simulink model "LQR_K_controller"  (R2017b)
settings: Solver=FixedStepAuto  StartTime=0.0  StopTime=inf  RelTol=1e-3
InitFcn:
  | set_kgain_from_physical_model_constraints
undefined symbols (not defined in the file or in its folder): Theta, X, Y
libraries: robotlib x17
settings Model: Creator=apollo  LastModifiedBy=apollo
settings OptimizationCC: PassReuseOutputArgsAs=Individual arguments  MaxStackSize=64
settings DebuggingCC: ParameterTunabilityLossMsg=error
settings HardwareCC: ProdBitPerPointer=32  ProdBitPerSizeT=32  ProdBitPerPtrDiffT=32  ProdLargestAtomicFloat=None  ProdIntDivRoundTo=Undefined  ProdEndianess=Unspecified  ProdWordSize=32  ProdHWDeviceType=Generic->Unspecified (assume 32-bit Generic)  UseEmbeddedCoderFeatures=off
settings SFSimCC: MATLABDynamicMemAlloc=off
settings RTWCC: SystemTargetFile=ert.tlc  HardwareBoard=Robot Operating System (ROS)  GenCodeOnly=on  TemplateMakefile=ert_default_tmf  GenerateReport=on  Toolchain=Catkin  IncludeHyperlinkInReport=on  LaunchReport=on  TargetLang=C++  GenerateTraceInfo=on  GenerateTraceReport=on  GenerateTraceReportSl=on  GenerateTraceReportSf=on  GenerateTraceReportEml=on
settings CodeAppCC: ForceParamTrailComments=on  IgnoreCustomStorageClasses=off  OperatorAnnotations=on  SimulinkDataObjDesc=on  SFDataObjDesc=on  InsertBlockDesc=on
settings ERTTargetCC: SupportNonInlinedSFcns=on

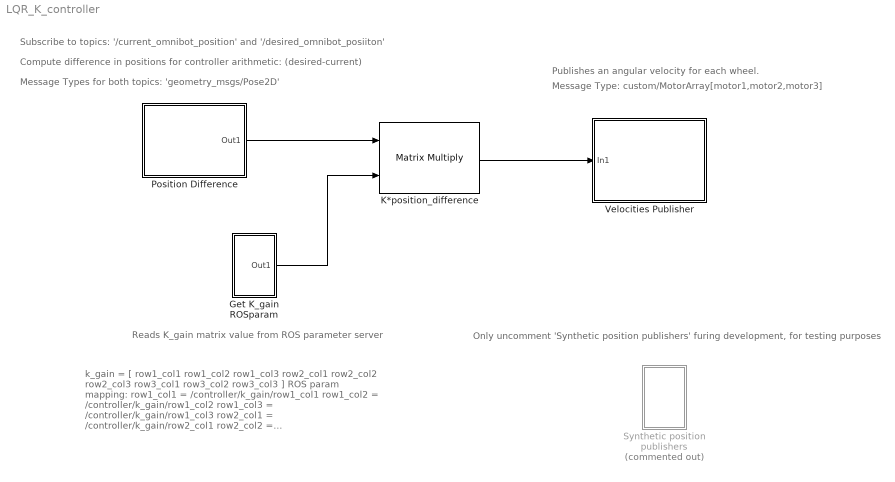
== system LQR_K_controller ==
  note: k_gain = [
      | row1_col1 row1_col2 row1_col3
      | row2_col1 row2_col2 row2_col3
      | row3_col1 row3_col2 row3_col3
      | ]
      |
      | ROS param mapping:
      | row1_col1 = /controller/k_gain/row1_col1
      | row1_col2 = /controller/k_gain/row1_col2
      | row1_col3 = /controller/k_gain/row1_col3
      |
      | row2_col1 = /controller/k_gain/row2_col1
      | row2_col2 = /controller/k_gain/row2_col2
      | row2_col3 = controller/k_gain/row2_col3
      |
      | row3_col1 = /controller/k_gain/row3_col1
      | row3_col2 = /controller/k_gain/row3_col2
      | row3_col3 = /controller/k_gain/row3_col3
  note: Reads K_gain matrix value from ROS parameter server
  note: Publishes an angular velocity for each wheel.
  note: Subscribe to topics: '/current_omnibot_position' and '/desired_omnibot_posiiton'
  note: Only uncomment 'Synthetic position publishers' furing development, for testing purposes
  note: Compute difference in positions for controller arithmetic: (desired-current)
  note: Message Types for both topics: 'geometry_msgs/Pose2D'
  note: Message Type: custom/MotorArray[motor1,motor2,motor3]
  Get K_gain ROSparam : Subsystem
  K*position_difference : Product  Multiplication=Matrix(*)
  Position Difference : Subsystem
  Synthetic position publishers : Subsystem  Commented=on
  Velocities Publisher : Subsystem
  wires:
  K*position_difference/1 -> Velocities Publisher/1(In1)
  Position Difference/1(Out1) -> K*position_difference/1
  Get K_gain ROSparam/1(Out1) -> K*position_difference/2

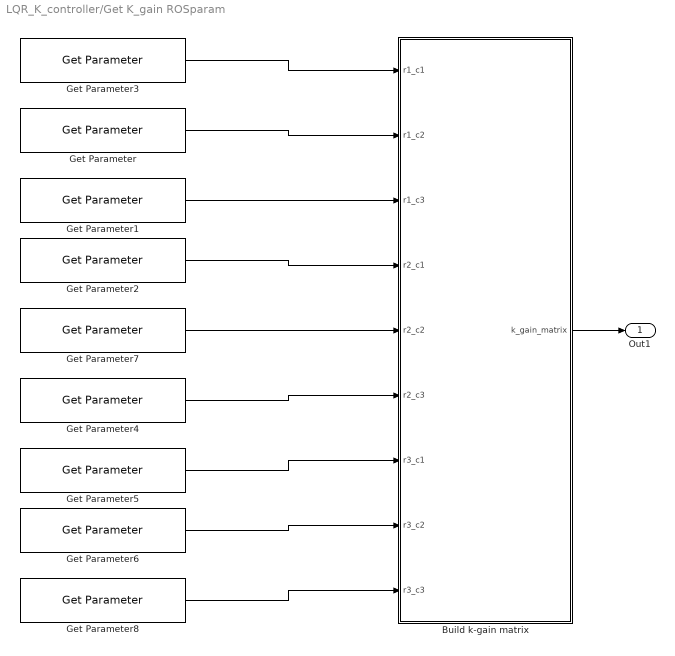
== system LQR_K_controller/Get K_gain ROSparam ==
  Build k-gain matrix : MATLAB Function  TreatAsAtomicUnit=on
  Get Parameter : robotlib/Get Parameter  SourceLibraryInfo=This block requires Robotics System Toolbox  ParameterSource=Specify your own  ParameterName=/controller/k_gain/row1_col2  ParameterType=double  ParameterMaxArrayLength=16  ParameterInitialValue=0.0  SampleTime=-1  ShowErrorCodeOutput=off  ModelName=LQR_K_controller  BlockId=ParamGet_LQR_K_controller_91
      settings: SourceProductName=Robotics System Toolbox  SourceProductBaseCode=RO
  Get Parameter1 : robotlib/Get Parameter  SourceLibraryInfo=This block requires Robotics System Toolbox  ParameterSource=Specify your own  ParameterName=/controller/k_gain/row1_col3  ParameterType=double  ParameterMaxArrayLength=16  ParameterInitialValue=0.0  SampleTime=-1  ShowErrorCodeOutput=off  ModelName=LQR_K_controller  BlockId=ParamGet_LQR_K_controller_92
      settings: SourceProductName=Robotics System Toolbox  SourceProductBaseCode=RO
  Get Parameter2 : robotlib/Get Parameter  SourceLibraryInfo=This block requires Robotics System Toolbox  ParameterSource=Specify your own  ParameterName=/controller/k_gain/row2_col1  ParameterType=double  ParameterMaxArrayLength=16  ParameterInitialValue=0.0  SampleTime=-1  ShowErrorCodeOutput=off  ModelName=LQR_K_controller  BlockId=ParamGet_LQR_K_controller_93
      settings: SourceProductName=Robotics System Toolbox  SourceProductBaseCode=RO
  Get Parameter3 : robotlib/Get Parameter  SourceLibraryInfo=This block requires Robotics System Toolbox  ParameterSource=Specify your own  ParameterName=/controller/k_gain/row1_col1  ParameterType=double  ParameterMaxArrayLength=16  ParameterInitialValue=0.0  SampleTime=-1  ShowErrorCodeOutput=off  ModelName=LQR_K_controller  BlockId=ParamGet_LQR_K_controller_94
      settings: SourceProductName=Robotics System Toolbox  SourceProductBaseCode=RO
  Get Parameter4 : robotlib/Get Parameter  SourceLibraryInfo=This block requires Robotics System Toolbox  ParameterSource=Specify your own  ParameterName=/controller/k_gain/row2_col3  ParameterType=double  ParameterMaxArrayLength=16  ParameterInitialValue=0.0  SampleTime=-1  ShowErrorCodeOutput=off  ModelName=LQR_K_controller  BlockId=ParamGet_LQR_K_controller_95
      settings: SourceProductName=Robotics System Toolbox  SourceProductBaseCode=RO
  Get Parameter5 : robotlib/Get Parameter  SourceLibraryInfo=This block requires Robotics System Toolbox  ParameterSource=Specify your own  ParameterName=/controller/k_gain/row3_col1  ParameterType=double  ParameterMaxArrayLength=16  ParameterInitialValue=0.0  SampleTime=-1  ShowErrorCodeOutput=off  ModelName=LQR_K_controller  BlockId=ParamGet_LQR_K_controller_96
      settings: SourceProductName=Robotics System Toolbox  SourceProductBaseCode=RO
  Get Parameter6 : robotlib/Get Parameter  SourceLibraryInfo=This block requires Robotics System Toolbox  ParameterSource=Specify your own  ParameterName=/controller/k_gain/row3_col2  ParameterType=double  ParameterMaxArrayLength=16  ParameterInitialValue=0.0  SampleTime=-1  ShowErrorCodeOutput=off  ModelName=LQR_K_controller  BlockId=ParamGet_LQR_K_controller_97
      settings: SourceProductName=Robotics System Toolbox  SourceProductBaseCode=RO
  Get Parameter7 : robotlib/Get Parameter  SourceLibraryInfo=This block requires Robotics System Toolbox  ParameterSource=Specify your own  ParameterName=/controller/k_gain/row2_col2  ParameterType=double  ParameterMaxArrayLength=16  ParameterInitialValue=0.0  SampleTime=-1  ShowErrorCodeOutput=off  ModelName=LQR_K_controller  BlockId=ParamGet_LQR_K_controller_98
      settings: SourceProductName=Robotics System Toolbox  SourceProductBaseCode=RO
  Get Parameter8 : robotlib/Get Parameter  SourceLibraryInfo=This block requires Robotics System Toolbox  ParameterSource=Specify your own  ParameterName=/controller/k_gain/row3_col3  ParameterType=double  ParameterMaxArrayLength=16  ParameterInitialValue=0.0  SampleTime=-1  ShowErrorCodeOutput=off  ModelName=LQR_K_controller  BlockId=ParamGet_LQR_K_controller_99
      settings: SourceProductName=Robotics System Toolbox  SourceProductBaseCode=RO
  Out1 : Outport
  wires:
  Get Parameter4/1 -> Build k-gain matrix/6(r2_c3)
  Get Parameter3/1 -> Build k-gain matrix/1(r1_c1)
  Get Parameter/1 -> Build k-gain matrix/2(r1_c2)
  Build k-gain matrix/1(k_gain_matrix) -> Out1/1
  Get Parameter2/1 -> Build k-gain matrix/4(r2_c1)
  Get Parameter7/1 -> Build k-gain matrix/5(r2_c2)
  Get Parameter8/1 -> Build k-gain matrix/9(r3_c3)
  Get Parameter6/1 -> Build k-gain matrix/8(r3_c2)
  Get Parameter5/1 -> Build k-gain matrix/7(r3_c1)
  Get Parameter1/1 -> Build k-gain matrix/3(r1_c3)

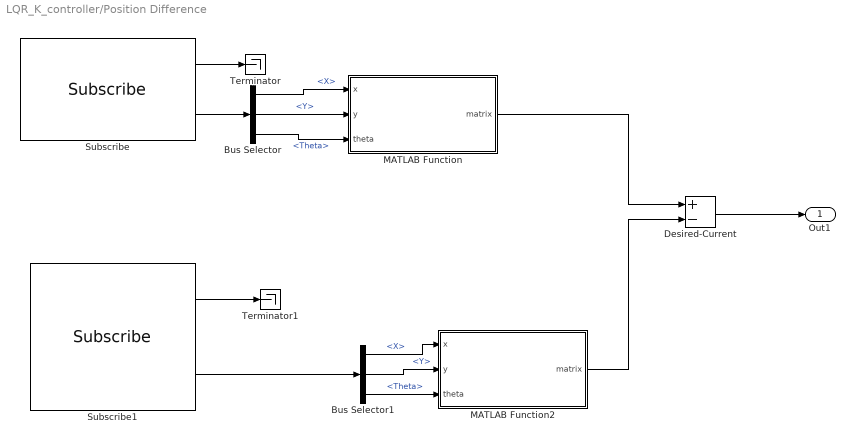
== system LQR_K_controller/Position Difference ==
  Bus Selector : BusSelector  OutputSignals=X,Y,Theta
  Bus Selector1 : BusSelector  OutputSignals=X,Y,Theta
  Desired-Current : Sum  Inputs=+-
  MATLAB Function : MATLAB Function  TreatAsAtomicUnit=on
  MATLAB Function2 : MATLAB Function  TreatAsAtomicUnit=on
  Subscribe : robotlib/Subscribe  SourceLibraryInfo=This block requires Robotics System Toolbox  topicSource=Specify your own  topic=/desired_omnibot_position  messageType=geometry_msgs/Pose2D  sampleTime=-1  messageQueueLength=1
      settings: SourceProductBaseCode=RO
  Subscribe1 : robotlib/Subscribe  SourceLibraryInfo=This block requires Robotics System Toolbox  topicSource=Specify your own  topic=/current_omnibot_position  messageType=geometry_msgs/Pose2D  sampleTime=-1  messageQueueLength=1
      settings: SourceProductBaseCode=RO
  Terminator : Terminator
  Terminator1 : Terminator
  Out1 : Outport
  wires:
  Subscribe/1 -> Terminator/1
  Subscribe1/1 -> Terminator1/1
  Subscribe/2 -> Bus Selector/1
  Bus Selector1/3 -> MATLAB Function2/3(theta)  "<Theta>"
  Bus Selector1/1 -> MATLAB Function2/1(x)  "<X>"
  Bus Selector1/2 -> MATLAB Function2/2(y)  "<Y>"
  Subscribe1/2 -> Bus Selector1/1
  MATLAB Function/1(matrix) -> Desired-Current/1
  Bus Selector/2 -> MATLAB Function/2(y)  "<Y>"
  Bus Selector/1 -> MATLAB Function/1(x)  "<X>"
  Bus Selector/3 -> MATLAB Function/3(theta)  "<Theta>"
  MATLAB Function2/1(matrix) -> Desired-Current/2
  Desired-Current/1 -> Out1/1

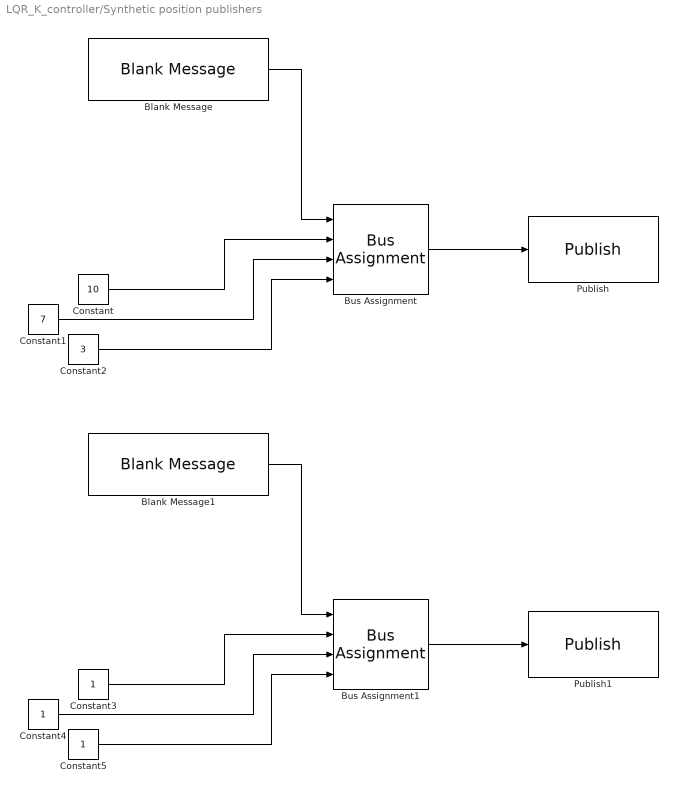
== system LQR_K_controller/Synthetic position publishers ==
  Blank Message : robotlib/Blank Message  SourceLibraryInfo=This block requires Robotics System Toolbox  messageType=geometry_msgs/Pose2D  SampleTime=inf
      settings: SourceProductBaseCode=RO
  Blank Message1 : robotlib/Blank Message  SourceLibraryInfo=This block requires Robotics System Toolbox  messageType=geometry_msgs/Pose2D  SampleTime=inf
      settings: SourceProductBaseCode=RO
  Bus Assignment : BusAssignment  AssignedSignals=X,Y,Theta
  Bus Assignment1 : BusAssignment  AssignedSignals=X,Y,Theta
  Constant : Constant  Value=10
  Constant1 : Constant  Value=7
  Constant2 : Constant  Value=3
  Constant3 : Constant
  Constant4 : Constant
  Constant5 : Constant
  Publish : robotlib/Publish  SourceLibraryInfo=This block requires Robotics System Toolbox  topicSource=Specify your own  topic=/current_omnibot_position  messageType=geometry_msgs/Pose2D  messageQueueLength=1
      settings: SourceProductBaseCode=RO
  Publish1 : robotlib/Publish  SourceLibraryInfo=This block requires Robotics System Toolbox  topicSource=Specify your own  topic=/desired_omnibot_position  messageType=geometry_msgs/Pose2D  messageQueueLength=1
      settings: SourceProductBaseCode=RO
  wires:
  Constant5/1 -> Bus Assignment1/4
  Bus Assignment1/1 -> Publish1/1
  Constant4/1 -> Bus Assignment1/3
  Blank Message/1 -> Bus Assignment/1
  Constant1/1 -> Bus Assignment/3
  Constant/1 -> Bus Assignment/2
  Bus Assignment/1 -> Publish/1
  Constant2/1 -> Bus Assignment/4
  Blank Message1/1 -> Bus Assignment1/1
  Constant3/1 -> Bus Assignment1/2

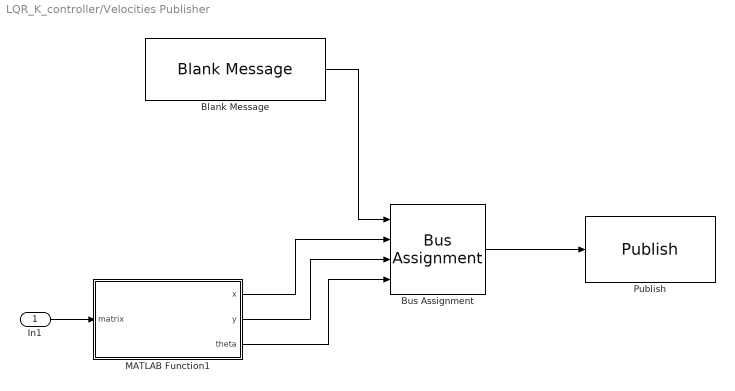
== system LQR_K_controller/Velocities Publisher ==
  In1 : Inport
  Blank Message : robotlib/Blank Message  SourceLibraryInfo=This block requires Robotics System Toolbox  messageType=geometry_msgs/Pose2D  SampleTime=inf
      settings: SourceProductBaseCode=RO
  Bus Assignment : BusAssignment  AssignedSignals=X,Y,Theta
  MATLAB Function1 : MATLAB Function  TreatAsAtomicUnit=on
  Publish : robotlib/Publish  SourceLibraryInfo=This block requires Robotics System Toolbox  topicSource=Specify your own  topic=/desired_velocities  messageType=geometry_msgs/Pose2D  messageQueueLength=1
      settings: SourceProductBaseCode=RO
  wires:
  In1/1 -> MATLAB Function1/1(matrix)
  Blank Message/1 -> Bus Assignment/1
  MATLAB Function1/1(x) -> Bus Assignment/2
  MATLAB Function1/2(y) -> Bus Assignment/3
  MATLAB Function1/3(theta) -> Bus Assignment/4
  Bus Assignment/1 -> Publish/1

== matlab function LQR_K_controller/Velocities Publisher/MATLAB Function1 ==
  data: matrix input; x output; y output; theta output
function [x, y, theta] = decompose_matrix(matrix)
    x = matrix(1);
    y = matrix(2);
    theta = matrix(3);
end

== matlab function LQR_K_controller/Position Difference/MATLAB Function ==
  data: x input; matrix output; y input; theta input
function matrix = compose_matrix(x,y,theta)
    matrix = [x y theta];
end

== matlab function LQR_K_controller/Position Difference/MATLAB Function2 ==
  data: x input; matrix output; y input; theta input
function matrix = compose_matrix(x,y,theta)
    matrix = [x y theta];
end

== matlab function LQR_K_controller/Get K_gain ROSparam/Build k-gain matrix ==
  data: r1_c1 input; k_gain_matrix output; r1_c2 input; r1_c3 input; r2_c1 input; r2_c2 input; r2_c3 input; r3_c1 input; r3_c2 input; r3_c3 input
function k_gain_matrix  = build_kgain_matrix(r1_c1,r1_c2,r1_c3,r2_c1,r2_c2,r2_c3,r3_c1,r3_c2,r3_c3)

k_gain_matrix = [
    r1_c1 r1_c2 r1_c3;
    r2_c1 r2_c2 r2_c3; 
    r3_c1 r3_c2 r3_c3
];
